simulink model "power_V2G_GA"  (R2015a)
settings: Solver=ode23tb  SolverMode=SingleTasking  StartTime=0.0  StopTime=24*60*60  RelTol=1e-4  AbsTol=1e-2
PreLoadFcn:
  | % Load Data and Parameters used by the model:
  | load power_V2G.mat
  | to=0.1;
undefined symbols (not defined in the file or in its folder): A, B, C, D1, Dd, Delta, Init, j, V2G
libraries: powerlib x54, simulink x19, simulink_extras x6, sps_avr x1, V2Glib x1, powerlib_meascontrol x1
(part 1 of 3)
Description:
  | Copyright 2008-2015 The MathWorks, Inc.
settings Model: SimulationMode=accelerator  CovSFcnEnable=off  ExtModeTrigDuration=100  Creator=MathWorks  LastModifiedBy=lenovo
settings SolverCC: MaxConsecutiveMinStep=1e6  ZeroCrossAlgorithm=Adaptive
settings OptimizationCC: BlockReduction=off  BooleanDataType=off
settings DebuggingCC: SaveWithParameterizedLinksMsg=none  UnderspecifiedInitializationDetection=Classic  MergeDetectMultiDrivingBlocksExec=none  SignalResolutionControl=TryResolveAllWithWarning
settings HardwareCC: TargetUnknown=on

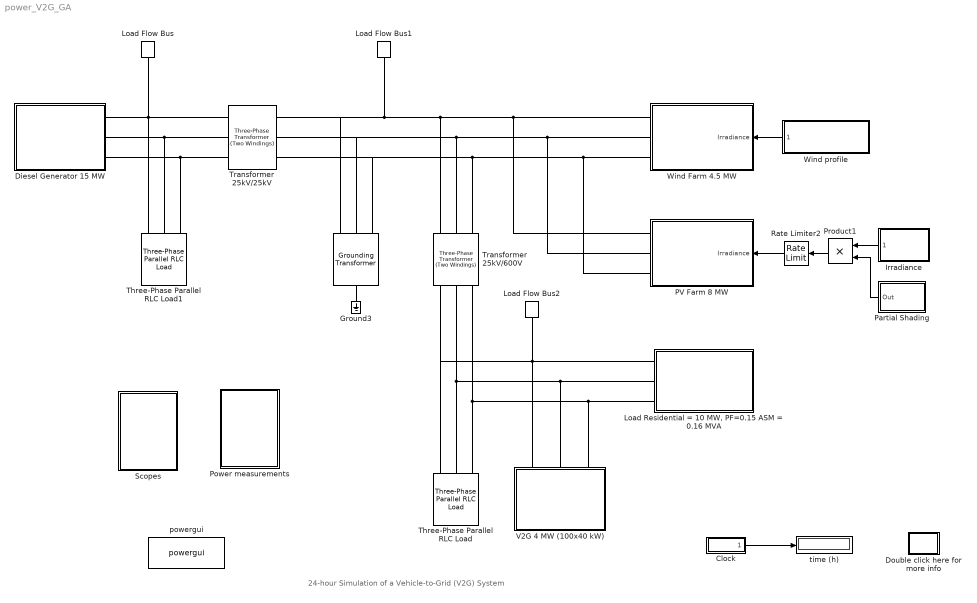
== system power_V2G_GA ==
  note: 24-hour Simulation of a Vehicle-to-Grid (V2G) System
  " " : powerlib/Elements/Grounding Transformer   UNITS=pu  NominalPower="[10e6   60]"  NominalVoltage=25e3  ZeroSequenceImpedance_pu=[0.00083333 9.4248]  MagnetizationBranch_pu=[5000 6283.2]  ZeroSequenceImpedance_SI=[0.25 7.5]  MagnetizationBranch_SI=[31250 31250]  Measurements=None
  Clock : Subsystem
  Diesel Generator 15 MW : Subsystem
      mask Display: image(imread('diesel.jpg'))
  Double click here for more info : Subsystem
      settings: OpenFcn=showdemo(bdroot(gcb))
      mask Display: disp('?')
  Ground3 : powerlib/Elements/Ground  LConnTagsString=a
  Irradiance : Subsystem
      mask init:
      | load power_V2G
      mask Display: plot(V2G.IRRADIANCE.time,V2G.IRRADIANCE.SUN)
  "Load Residential = 10 MW, PF=0.15 ASM = 0.16 MVA " : Subsystem
      mask Display: image(imread('load.jpg'))
  Load Flow Bus : powerlib/Measurements/Load Flow Bus  LConnTagsString=a  ID=BUS_1  Vbase=25e3  Vref=1  Vangle=0  VLF=1  angleLF=0
      settings: AttributesFormatString=%<ID>\n%<Vbase>V\n%<VLF>pu\n%<angleLF>deg.
  Load Flow Bus1 : powerlib/Measurements/Load Flow Bus  LConnTagsString=a  ID=BUS_2  Vbase=25e3  Vref=1  Vangle=0  VLF=0.9783  angleLF=-0.1322
      settings: AttributesFormatString=%<ID>\n%<Vbase>V\n%<VLF>pu\n%<angleLF>deg.
  Load Flow Bus2 : powerlib/Measurements/Load Flow Bus  LConnTagsString=a  ID=BUS_3  Vbase=1e3  Vref=1  Vangle=0  VLF=0.9583  angleLF=-3.174
      settings: AttributesFormatString=%<ID>\n%<Vbase>V\n%<VLF>pu\n%<angleLF>deg.
  PV Farm 8 MW : Subsystem  mask{eff=10, area=8e4}
      mask prompts: eff "Efficiency (%)"; area "Area (m^2)"
      mask help: The product of the effeciency, the area covered by the Pv farm and the irradiance in w/m2 will give you the power generate by the PV farm
      mask DialogControl DescGroupVar Prompt: PV farm
      mask DialogControl DescTextVar Prompt: The product of the efficiency, the area covered by the PV farm and the irradiance in W/m2 will give you the power generated by the PV farm.
      mask Display: image(imread('panel.jpg'))
  Partial Shading : Subsystem  mask(Signal Disturbance){Hour=12, Minute=0, Second=0, Duration=5*60, Factor=0.7}
      mask prompts: Duration "Duration (s):"
      mask help: Within the specified time range defined by Start and Duration parameters, output is set to 'Factor'. Outside the specified time range output is kept at 1.0.
      mask init:
      | T2=(Hour-1)*60*60;    % Hour in seconds
      | T3=(Minute-1)*60;  % Minute in seconds
      | Ton=T2+T3+(Second-1);    % Beginning of fault (s)
      | Toff=Ton+Duration; % End of fault (s)
      mask TypeOptions Hour: 0 |      1 |      2 |      3 |      4 |      5 |      6 |      7 |      8 |      9 |     10 |     11 |     12 |     13 |     14 |     15 |     16 |     17 |     18 |     19 |     20 |     21 |     22 |     23
      mask TypeOptions Minute: 0 |      1 |      2 |      3 |      4 |      5 |      6 |      7 |      8 |      9 |     10 |     11 |     12 |     13 |     14 |     15 |     16 |     17 |     18 |     19 |     20 |     21 |     22 |     23 |     24 |     25 |     26 |     27 |     28 |     29 |     30 |     31 |     32 |     33 |     34 |     35 |     36 |     37 |     38 |     39 |     40 |     41 |     42 |     43 |     44 |     45 |     46 |     47 |     48 |     49 |     50 |     51 |     52 |     53 |     54 |     55 |     56 |     57 |     58 |     59
      mask TypeOptions Second: 0 |      1 |      2 |      3 |      4 |      5 |      6 |      7 |      8 |      9 |     10 |     11 |     12 |     13 |     14 |     15 |     16 |     17 |     18 |     19 |     20 |     21 |     22 |     23 |     24 |     25 |     26 |     27 |     28 |     29 |     30 |     31 |     32 |     33 |     34 |     35 |     36 |     37 |     38 |     39 |     40 |     41 |     42 |     43 |     44 |     45 |     46 |     47 |     48 |     49 |     50 |     51 |     52 |     53 |     54 |     55 |     56 |     57 |     58 |     59
      mask DialogControl Control2 Prompt: Start:
  Power measurements : Subsystem
  Product1 : Product
  Rate Limiter2 : RateLimiter  RisingSlewLimit=1e4  FallingSlewLimit=-1e4  SampleTimeMode=inherited
  "Scopes " : Subsystem
  Three-Phase Parallel RLC Load : powerlib/Elements/Three-Phase Parallel RLC Load  LConnTagsString=A|B|C  Configuration=Y (grounded)  NominalVoltage=(1000)*0.958281  NominalFrequency=60  ActivePower=1e3  InductivePower=0  CapacitivePower=0  Measurements=None  LoadType=constant PQ
  Three-Phase Parallel RLC Load1 : powerlib/Elements/Three-Phase Parallel RLC Load  LConnTagsString=A|B|C  Configuration=Y (grounded)  NominalVoltage=(25000)*1  NominalFrequency=60  ActivePower=1e3  InductivePower=0  CapacitivePower=0  Measurements=None  LoadType=constant PQ
  Transformer 25kV/25kV : powerlib/Elements/Three-Phase Transformer (Two Windings)  Winding1Connection=Yg  Winding2Connection=Yg  CoreType=Three single-phase transformers  SetSaturation=off  Hysteresis=off  DataFile='hysteresis'  SetInitialFlux=off  Measurements=None  UNITS=pu  NominalPower=[ 20e6 , 60 ]  Winding1=[25e3 , 0.002 , 0.08 ]  Winding2=[ 25e3 , 0.002 , 0.08 ]  Rm=500  Lm=500  L0=0.5  Saturation=[ 0,0 ; 0.0024,1.2 ; 1.0,1.52 ]  InitialFluxes=[ 0.8 , -0.8 , 0.7 ]  MoreParameters=off  BreakLoop=off  DataType=off  TransfoNumber=1
  Transformer 25kV/600V : powerlib/Elements/Three-Phase Transformer (Two Windings)  Winding1Connection=Yg  Winding2Connection=Yg  CoreType=Three single-phase transformers  SetSaturation=off  Hysteresis=off  DataFile='hysteresis'  SetInitialFlux=off  Measurements=None  UNITS=pu  NominalPower=[ 20e6 , 60 ]  Winding1=[25e3 , 0.002 , 0.08 ]  Winding2=[ 600 , 0.002 , 0.08 ]  Rm=500  Lm=500  L0=0.5  Saturation=[ 0,0 ; 0.0024,1.2 ; 1.0,1.52 ]  InitialFluxes=[ 0.8 , -0.8 , 0.7 ]  MoreParameters=off  BreakLoop=off  DataType=off  TransfoNumber=1
  V2G 4 MW (100x40 kW) : Subsystem  mask{nomPower=20*2, capacity=85, eff=90, enable=on, regGain=[2 4e3], cars1=35, cars2=25, cars3=10, cars4=20, cars5=10}
      mask prompts: nomPower "Rated power (kW)"; capacity "Rated capacity (kWh)"; eff "System efficiency (%)"; enable "V2G on"; regGain "Regulator gain [Kp Ki]"; cars1 "Number of cars  (profile 1)"; cars2 "Number of cars  (profile 2)"; cars3 "Number of cars  (profile 3)"; cars4 "Number of cars  (profile 4)"; cars5 "Number of cars  (profile 5)"
      mask DialogControl DescGroupVar Prompt: V2G
      mask DialogControl DescTextVar Prompt: Models a generic aggregation of electric vehicles. The model has 5 different profiles that can be modified under the mask by changing the plug and the state of charge lookup tables of each profile. The user can set the number of vehicles following each type of profile. The rated capacity, the rated power and the efficiency of the power converter can also be decided by the user. See the example documentation for information about various user profiles.
      mask Display: image(imread('EV.jpg'))
  Wind Farm 4.5 MW : Subsystem  mask{nomPower=4.5, nomwind=13.5, maxwind=15}
      mask prompts: nomPower "Nominal power (MW)"; nomwind "Nominal wind speed (m/s)"; maxwind "Maximal wind speed (m/s)"
      mask DialogControl DescGroupVar Prompt: Wind farm
      mask DialogControl DescTextVar Prompt: The simplified wind farm model presented here generates power using a linear relationship between the nominal wind speed and nominal power. When the wind speed reaches the maximal value, the wind farm trips from the grid. When the wind speed is between the nominal speed and the maximal value, the power is fixed to 1 p.u.
      mask Display: image(imread('windfarm.jpg'))
  Wind profile : Subsystem
      mask init:
      | load power_V2G
      mask Display: plot(V2G.WINDTURBINE.time,V2G.WINDTURBINE.wind)
  powergui : powerlib/powergui  Priority=1  SimulationMode=Phasor  SolverType=Tustin  SampleTime=50e-6  frequency=60  SPID=off  DisableSnubberDevices=off  DisableRonSwitches=off  DisableVfSwitches=off  SwTol=0  DisplayEquations=off  Interpol=off  methode=off  Ts=100  FunctionMessages=off  echomessages=off  HookPort=off  EnableUseOfTLC=off  x0status=blocks  frequencyindice=60  Pbase=10e6  ErrMax=0.0001  Iterations=50  UnitsV=kV  UnitsW=MW  buscounter=0  RestoreLinks=warning  ResistiveCurrentMeasurement=off  Frange=[0:2:500]  Ylog=off  Xlog=on  ShowGrid=off  save=off  variable=ZData  structure=0  ZoomFFT=off  StartTime=0.0  cycles=1  DisplayStyle=1  fundamental=60  FreqAxis=off  MaxFrequency=1000  frequencyindicesteady=1  RmsSteady=1  display=off
  time (h) : Display
      settings: Format=bank
  wires:
  Irradiance/1(" ") -> Product1/1
  Product1/1 -> Rate Limiter2/1
  Wind profile/1(" ") -> Wind Farm 4.5 MW/1(Irradiance)
  Partial Shading/1(Out) -> Product1/2
  Rate Limiter2/1 -> PV Farm 8 MW/1(Irradiance)
  Clock/1(" ") -> time (h)/1
  connections:
  "Load Residential = 10 MW, PF=0.15 ASM = 0.16 MVA "/LConn3 -- V2G 4 MW (100x40 kW)/LConn3 -- Three-Phase Parallel RLC Load/LConn3 -- Transformer 25kV/600V/RConn3
  Transformer 25kV/600V/LConn3 -- " "/LConn3 -- Transformer 25kV/25kV/RConn3 -- PV Farm 8 MW/RConn3 -- Wind Farm 4.5 MW/RConn3
  " "/RConn1 -- Ground3/LConn1
  Load Flow Bus/LConn1 -- Transformer 25kV/25kV/LConn1 -- Diesel Generator 15 MW/RConn1 -- Three-Phase Parallel RLC Load1/LConn1
  "Load Residential = 10 MW, PF=0.15 ASM = 0.16 MVA "/LConn1 -- Load Flow Bus2/LConn1 -- V2G 4 MW (100x40 kW)/LConn1 -- Three-Phase Parallel RLC Load/LConn1 -- Transformer 25kV/600V/RConn1
  "Load Residential = 10 MW, PF=0.15 ASM = 0.16 MVA "/LConn2 -- V2G 4 MW (100x40 kW)/LConn2 -- Three-Phase Parallel RLC Load/LConn2 -- Transformer 25kV/600V/RConn2
  Transformer 25kV/600V/LConn1 -- Transformer 25kV/25kV/RConn1 -- " "/LConn1 -- Load Flow Bus1/LConn1 -- Wind Farm 4.5 MW/RConn1 -- PV Farm 8 MW/RConn1
  Transformer 25kV/600V/LConn2 -- " "/LConn2 -- Transformer 25kV/25kV/RConn2 -- PV Farm 8 MW/RConn2 -- Wind Farm 4.5 MW/RConn2
  Transformer 25kV/25kV/LConn3 -- Diesel Generator 15 MW/RConn3 -- Three-Phase Parallel RLC Load1/LConn3
  Transformer 25kV/25kV/LConn2 -- Diesel Generator 15 MW/RConn2 -- Three-Phase Parallel RLC Load1/LConn2

== system power_V2G_GA/Clock ==
  Clock : Clock
  Gain : Gain  Gain=1/(60*60)
  " " : Outport
  wires:
  Gain/1 -> " "/1
  Clock/1 -> Gain/1

== system power_V2G_GA/Diesel Generator 15 MW ==
  " Load Measurements" : powerlib/Measurements/Three-Phase V-I Measurement  VoltageMeasurement=phase-to-ground  SetLabelV=on  LabelV=Vabc1  Vpu=off  VpuLL=off  CurrentMeasurement=yes  SetLabelI=on  LabelI=Iabc1  Ipu=off  Pbase=2*1.5e6/0.9  Vbase=25e3  OutputType=Complex  PhasorSimulation=on  PSBequivalent=0
  Bus Selector : BusSelector  OutputSignals="dq0 components.Stator voltage  vq (pu),dq0 components.Stator voltage  vd (pu),Mechanical.Rotor speed  wm  (pu)"
  Constant1 : Constant
  Constant2 : Constant
  Diesel Engine Governor : Subsystem  mask(Diesel Engine & Governor){K=29, Tr=[0.01 0.02 0.2], Ta=[0.25 0.009 0.0384], Tlim=[0 1.1], Td=0.024, Pm0=0.1361}
      mask prompts: K "Regulator gain K:"; Tr "Regulator time constants [T1 T2 T3 ] (s) :"; Ta "Actuator time constants [T4 T5 T6] (s) :"; Tlim "Torque limits [Tmin Tmax] (pu) :"; Td "Engine time delay Td (s) :"; Pm0 "Initial value of mechanical power  Pm0 (pu) :"
      mask help:
      | This block implements a diesel engine and governor system:
      | 1st and 2nd inputs: Desired and actual speed (pu)
      | Output: Diesel engine mechanical power.Motor inertia should be combined with generator.
      | Controller transfer function:
      |      Hc=K.(1+T3.s)/(1+T1.s+T1.T2.s^2)
      | Actuator transfer function :
      |      Ha= (1+T4.s) / [ (s (1+T5.s)(1+T6.s) ]
      | Motor :
      |      Time delay Td
      |
      | (See reference in Tutorial Session 5)
  Excitation System : sps_avr/Excitation System  tr=20e-3  reg=[ 300, 0.001 ]  exc=[ 1, 0 ]  tgr=[ 0, 0 ]  damp=[ 0.001, 0.1 ]  sat=[ 0, 0 ]  lim=[ -11.5, 11.5, 0 ]  v0=[1 1.2473]
  Ground : Ground
  Rotor speed (p.u.) : Scope
      settings: TimeRange=86400  YMin=0.9955  YMax=1.005  SaveName=wm1
  Synchronous Machine pu Standard : powerlib/Machines/Synchronous Machine pu Standard  PresetModel=No  MechanicalLoad=Mechanical power Pm  ShowDetailedParameters=on  RotorType=Salient-pole  Units=per unit standard parameters  MeasurementBus=off  NominalParameters="[ 15E6  25e3   60]"  Reactances1=[ 1.81, 0.3, 0.23, 1.76, 0.65, 0.25, 0.15 ]  Reactances2="[ 1.305, 0.296, 0.252, 0.474,  0.243,  0.18 ]"  dAxisTimeConstants=Open-circuit  qAxisTimeConstants=Short-circuit  TimeConstants1="[ 4.4849  0.0681  0.1  ]"  TimeConstants2=[ 8.0, 0.03, 1.0, 0.07 ]  TimeConstants3="[  4.49  0.0681  0.0513  ]"  TimeConstants4=[ 8.0, 0.03, 0.3371, 0.0295 ]  TimeConstants5=[ 1.01, 0.053, 0.1 ]  TimeConstants6=[ 1.3201, 0.023, 1.0, 0.07 ]  TimeConstants7=[0.012 0.003 0.003]  TimeConstants8=[ 1.3201, 0.0231, 0.3371, 0.0295 ]  StatorResistance=0.003  Mechanical=[3.7 0 1 ]  PolePairs=20  InitialConditions=[0 -86.6365 0.2279 0.2279 0.2279 -53.3785 -173.379 66.6215 1.24735]  SetSaturation=off  Saturation=[0.6404,0.7127,0.8441,0.9214,0.9956,1.082,1.19,1.316,1.457;0.7,0.7698,0.8872,0.9466,0.9969,1.046,1.1,1.151,1.201]  LoadFlowParameters=[1,0,0,0,0]  TsPowergui=0  TsBlock=-1  IterativeModel=Trapezoidal non iterative  BusType=swing  Pref=0  Qref=0  Qmin=-inf  Qmax=inf  PLF=0  QLF=0
  A : PMIOPort  Port=1  Side=Right
  B : PMIOPort  Port=2  Side=Right
  C : PMIOPort  Port=3  Side=Right
  tag scope: wm=global
  wires:
  Bus Selector/3 -> Diesel Engine Governor/2(w (pu)), Rotor speed (p.u.)/1, [wm]  "<Rotor speed  wm  (pu)>"
  Constant1/1 -> Diesel Engine Governor/1(wref (pu))
  Diesel Engine Governor/1(Pmec (pu)) -> Synchronous Machine pu Standard/1
  Excitation System/1 -> Synchronous Machine pu Standard/2
  Constant2/1 -> Excitation System/1
  Bus Selector/2 -> Excitation System/2  "<Stator voltage  vd (pu)>"
  Bus Selector/1 -> Excitation System/3  "<Stator voltage  vq (pu)>"
  Synchronous Machine pu Standard/1 -> Bus Selector/1
  Ground/1 -> Excitation System/4
  connections:
  " Load Measurements"/RConn1 -- A/RConn1
  C/RConn1 -- " Load Measurements"/RConn3
  B/RConn1 -- " Load Measurements"/RConn2
  Synchronous Machine pu Standard/RConn3 -- " Load Measurements"/LConn3
  Synchronous Machine pu Standard/RConn2 -- " Load Measurements"/LConn2
  Synchronous Machine pu Standard/RConn1 -- " Load Measurements"/LConn1

== system power_V2G_GA/Double click here for more info ==

== system power_V2G_GA/Irradiance ==
  1-D Lookup IRRADIANCE Table : Lookup_n-D  NumberOfTableDimensions=1  BreakpointsForDimension1=V2G.IRRADIANCE.time  BeginIndexSearchUsingPreviousIndexResult=on  Table=V2G.IRRADIANCE.SUN  InternalRulePriority=Speed  RndMeth=Simplest  InputSameDT=on
  Add : Sum
  Clock : Clock
  Constant1 : Constant
  Second-->Hour : Gain  Gain=1/(60*60)
  " " : Outport
  wires:
  Constant1/1 -> Add/2
  Add/1 -> 1-D Lookup IRRADIANCE Table/1  "Hour of the day"
  1-D Lookup IRRADIANCE Table/1 -> " "/1
  Clock/1 -> Second-->Hour/1
  Second-->Hour/1 -> Add/1

== system power_V2G_GA/Load Residential = 10 MW, PF=0.15 ASM = 0.16 MVA  ==
  " ASM Measurements" : powerlib/Measurements/Three-Phase V-I Measurement  VoltageMeasurement=phase-to-ground  SetLabelV=on  LabelV=Vasm  Vpu=off  VpuLL=off  CurrentMeasurement=yes  SetLabelI=on  LabelI=Iasm  Ipu=off  Pbase=2*1.5e6/0.9  Vbase=25e3  OutputType=Complex  PhasorSimulation=on  PSBequivalent=0
  " Load Measurements" : powerlib/Measurements/Three-Phase V-I Measurement  VoltageMeasurement=phase-to-ground  SetLabelV=on  LabelV=Vload  Vpu=off  VpuLL=off  CurrentMeasurement=yes  SetLabelI=on  LabelI=Iload  Ipu=off  Pbase=2*1.5e6/0.9  Vbase=25e3  OutputType=Complex  PhasorSimulation=on  PSBequivalent=0
  Asynchronous Machine (customized) : V2Glib/Asynchronous Machine (custom)  RotorType=Squirrel-cage  PresetModel=No  MechanicalLoad=Torque Tm  ShowDetailedParameters=on  ReferenceFrame=Rotor  Units=pu  MeasurementBus=on  NominalParameters=[1.5e+05 600 60]  Stator=[0.01117 0.04832]  Rotor=[0.006 0.04832]  Cage1=[0.01909 0.0397]  Cage2=[0.01909 0.0397]  Lm=2.424  Mechanical=[0.3096 0.01511 2]  PolePairs=2  InitialConditions=[1 0 0 0 0 0 0 0]  SimulateSaturation=off  Saturation="[0.212,0.4201,0.8125,1.0979,1.4799,2.2457,3.2586,4.5763,6.4763 ;   0.5,0.7,0.9,1,1.1,1.2 ,1.3,1.4,1.5]"  LoadFlowParameters=0  TsPowergui=0  TsBlock=-1  IterativeModel=Trapezoidal non iterative  Pmec=2e6
  Gain : Gain  Gain=1.492e5
  Gain1 : Gain  Gain=1.018/(0.9825^2)
  Math Function : Math  Operator=square  SaturateOnIntegerOverflow=on
  P electric : Display
  Product : Product
  Rate Limiter2 : RateLimiter  RisingSlewLimit=1e4  FallingSlewLimit=-1e4  SampleTimeMode=inherited
  Residential Load : Subsystem  mask{nomPower=10, PF=0.95, timestep=60, datas=V2G.CONSUMPTION}
      mask prompts: nomPower "Nominal Power (MW)"; PF "Power factor"; timestep "Timestep (minutes)"; datas "Consumption datas"
      mask DialogControl DescGroupVar Prompt: Load profile
      mask DialogControl DescTextVar Prompt: The load profile allows you to fix a nominal power and and a power factor. It is also needed to specify the timestep used for the consumption datas. Finally, a vector expresses the consumption profile. It has to be expressed in per unit. It is imperative that the length of the vector fits with the timestep used.
      mask Display: image(imread('Residential.jpg'))
  Rotor speed (p.u.) : Display
  Te(p.u.) : Display
  Three-Phase Breaker2 : powerlib/Elements/Three-Phase Breaker  InitialState=open  SwitchA=on  SwitchB=on  SwitchC=on  SwitchTimes=[ 3*3600]  External=off  BreakerResistance=0.001  SnubberResistance=1e6  SnubberCapacitance=inf  Measurements=None
  Three-Phase Fault : powerlib/Elements/Three-Phase Fault  InitialStates=0  FaultA=off  FaultB=off  FaultC=off  GroundFault=on  SwitchTimes=[4*3600 4*3600+100]  External=off  SwitchStatus=NaN  FaultResistance=0.001  GroundResistance=0.01  SnubberResistance=1e6  SnubberCapacitance=inf  Measurements=None
  A : PMIOPort  Port=1  Side=Left
  B : PMIOPort  Port=2  Side=Left
  C : PMIOPort  Port=3  Side=Left
  wires:
  Gain1/1 -> Rate Limiter2/1
  Asynchronous Machine (customized)/1 -> Rotor speed (p.u.)/1, Product/1, Math Function/1
  Asynchronous Machine (customized)/2 -> Product/2, Te(p.u.)/1
  Product/1 -> Gain/1
  Gain/1 -> P electric/1
  Rate Limiter2/1 -> Asynchronous Machine (customized)/1
  Math Function/1 -> Gain1/1
  connections:
  " Load Measurements"/LConn3 -- Residential Load/LConn3
  " Load Measurements"/LConn2 -- Residential Load/LConn2
  " Load Measurements"/LConn1 -- Residential Load/LConn1
  " ASM Measurements"/RConn2 -- " Load Measurements"/RConn2 -- B/RConn1
  " ASM Measurements"/RConn3 -- " Load Measurements"/RConn3 -- C/RConn1
  " Load Measurements"/RConn1 -- A/RConn1 -- " ASM Measurements"/RConn1
  Asynchronous Machine (customized)/LConn2 -- Three-Phase Fault/LConn2 -- Three-Phase Breaker2/LConn2
  Asynchronous Machine (customized)/LConn3 -- Three-Phase Breaker2/LConn3 -- Three-Phase Fault/LConn3
  Three-Phase Breaker2/RConn1 -- " ASM Measurements"/LConn1
  Three-Phase Breaker2/RConn2 -- " ASM Measurements"/LConn2
  Three-Phase Breaker2/RConn3 -- " ASM Measurements"/LConn3
  Three-Phase Breaker2/LConn1 -- Three-Phase Fault/LConn1 -- Asynchronous Machine (customized)/LConn1

== system power_V2G_GA/PV Farm 8 MW ==
  Irradiance : Inport
  Irradiance data : Subsystem
  PV Farm : Subsystem
  VabcPV : powerlib/Measurements/Three-Phase V-I Measurement  VoltageMeasurement=phase-to-ground  SetLabelV=on  LabelV=VabcPV  Vpu=off  VpuLL=off  CurrentMeasurement=yes  SetLabelI=on  LabelI=IabcPV  Ipu=off  Pbase=2*1.5e6/0.9  Vbase=25e3  OutputType=Complex  PhasorSimulation=on  PSBequivalent=0
  A : PMIOPort  Port=1  Side=Right
  B : PMIOPort  Port=2  Side=Right
  C : PMIOPort  Port=3  Side=Right
  wires:
  Irradiance data/1(Out1) -> PV Farm/1(P)
  Irradiance/1 -> Irradiance data/1("Data ")
  connections:
  B/RConn1 -- VabcPV/RConn2
  VabcPV/LConn2 -- PV Farm/RConn2
  A/RConn1 -- VabcPV/RConn1
  VabcPV/RConn3 -- C/RConn1
  PV Farm/RConn1 -- VabcPV/LConn1
  VabcPV/LConn3 -- PV Farm/RConn3

== system power_V2G_GA/Partial Shading ==
  Add : Sum
  Clock : Clock
  Compare To Constant : simulink/Logic and Bit Operations/Compare To Constant  relop=>=  const=Ton  OutDataTypeStr=boolean
  Compare To Constant1 : simulink/Logic and Bit Operations/Compare To Constant  relop=<  const=Toff  OutDataTypeStr=boolean
  Constant : Constant  Value=Factor
  Logical Operator : Logic  AllPortsSameDT=off  OutDataTypeStr=float('double')
  Logical Operator1 : Logic  Operator=NOT  AllPortsSameDT=off  OutDataTypeStr=float('double')
  Product : Product
  Out : Outport
  wires:
  Add/1 -> Out/1
  Product/1 -> Add/2
  Constant/1 -> Product/2
  Compare To Constant/1 -> Logical Operator/1
  Clock/1 -> Compare To Constant1/1, Compare To Constant/1
  Compare To Constant1/1 -> Logical Operator/2
  Logical Operator/1 -> Logical Operator1/1, Product/1
  Logical Operator1/1 -> Add/1

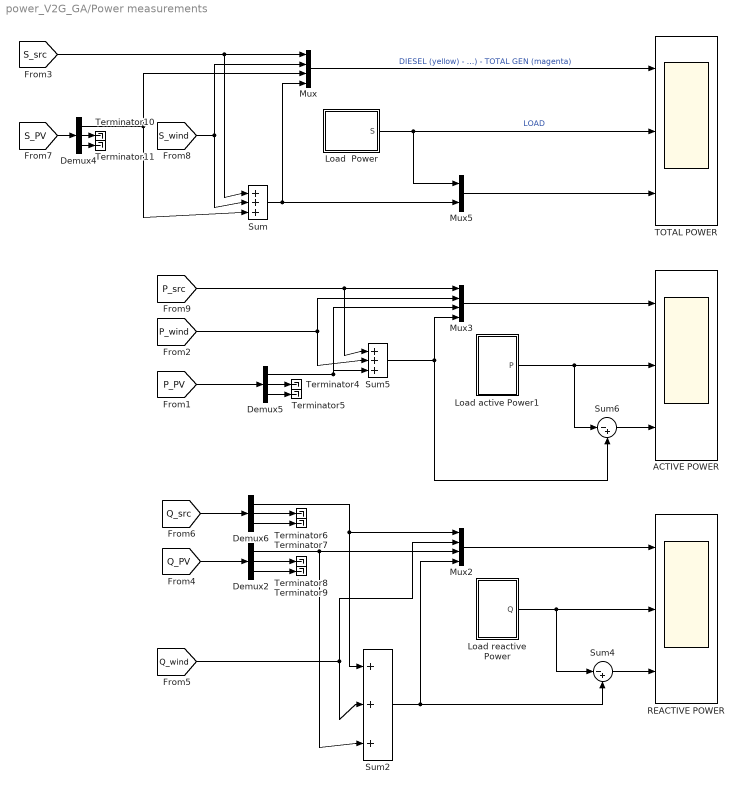
== system power_V2G_GA/Power measurements ==
  ACTIVE POWER : Scope  NumInputPorts=3
      settings: TimeRange=86394.68034477012  YMin=-1127645.502645526~0~0  YMax=14321145.12471653~14000000~194678.5071649832  SaveName=ScopeData9  Decimation=20
  Demux{2,4..6} (4 alike) : Demux  Outputs=3
  Load  Power : Subsystem
  Load active Power1 : Subsystem
  Load reactive Power : Subsystem
  Mux : Mux
  Mux2 : Mux
  Mux3 : Mux
  Mux5 : Mux  Inputs=2
  REACTIVE POWER : Scope  NumInputPorts=3
      settings: TimeRange=86394.68034477012  YMin=-639880.9523809515~29417.73813057679~0  YMax=7141203.703703707~4200987.36115234~2993413.800705456  SaveName=ScopeData7  Decimation=20
  Sum : Sum  Inputs=|+++
  Sum2 : Sum  Inputs=|+++
  Sum4 : Sum  Inputs=|-+
  Sum5 : Sum  Inputs=|+++
  Sum6 : Sum  Inputs=|-+
  TOTAL POWER : Scope  NumInputPorts=3
      settings: TimeRange=86395.43113750442  YMin=0~0~123381.0870346278  YMax=16020911.12187349~14000000~16409684.57560659  SaveName=ScopeData5  Decimation=20
  Terminator{4..11} (8 alike) : Terminator
  wires:
  [Q_src] -> Demux6/1
  [S_src] -> Sum/1, Mux/1
  [S_wind] -> Mux/2, Sum/2
  Sum/1 -> Mux/4, Mux5/2
  Demux6/1 -> Sum2/1, Mux2/1
  [Q_wind] -> Mux2/2, Sum2/2
  Sum2/1 -> Sum4/2, Mux2/4
  Mux/1 -> TOTAL POWER/1  "DIESEL (yellow) - WIND (red) - PV FARM (green) - TOTAL GEN (magenta)"
  Mux2/1 -> REACTIVE POWER/1
  Sum4/1 -> REACTIVE POWER/3
  Mux5/1 -> TOTAL POWER/3
  Load  Power/1(S) -> TOTAL POWER/2, Mux5/1  "LOAD"
  [Q_PV] -> Demux2/1
  Demux2/1 -> Sum2/3, Mux2/3
  [S_PV] -> Demux4/1
  Demux4/2 -> Terminator10/1
  Demux4/3 -> Terminator11/1
  Demux4/1 -> Mux/3, Sum/3
  Load reactive Power/1("Q ") -> Sum4/1, REACTIVE POWER/2
  [P_wind] -> Sum5/2, Mux3/2
  [P_src] -> Sum5/1, Mux3/1
  Sum5/1 -> Sum6/2, Mux3/4
  Mux3/1 -> ACTIVE POWER/1
  Load active Power1/1(P) -> Sum6/1, ACTIVE POWER/2
  Sum6/1 -> ACTIVE POWER/3
  [P_PV] -> Demux5/1
  Demux5/1 -> Sum5/3, Mux3/3
  Demux5/2 -> Terminator4/1
  Demux5/3 -> Terminator5/1
  Demux6/2 -> Terminator6/1
  Demux6/3 -> Terminator7/1
  Demux2/2 -> Terminator8/1
  Demux2/3 -> Terminator9/1

== system power_V2G_GA/Scopes  ==
  note: Scopes related to production
  note: Scopes related to the consumption
  note: Scopes related to the V2G system
  ASM : Scope  NumInputPorts=5
      settings: TimeRange=86394.68034477012  YMin=383.346641994195~0~0~-279310.3448275863~-231272.2948870416  YMax=518.2077387266461~464.9227110582633~270214.030915576~0~92152.19976218522  SaveName=ScopeData10  Decimation=20
  ASMdata : Subsystem
  Charge : Scope  NumInputPorts=5
      settings: YMin=449.78~0.00075~0.5~-0.95~-0.3  YMax=449.87~0.00135~0.95~-0.45~0.3  SaveName=ScopeData17  Decimation=20
  Charge data : Subsystem
  Load : Scope  NumInputPorts=5
      settings: TimeRange=86394.68034477012  YMin=395.7726844069046~6091.95402298851~4224137.931034483~-11810344.8275862~-4000000  YMax=499.0979539956536~18045.97701149426~12500000~-3706896.551724136~-655172.4137931094  Decimation=20
  "Load data " : Subsystem
  PV Farm : Scope  NumInputPorts=5
      settings: TimeRange=86394.68034477012  YMin=18282.00607471011~0~0~-124521.0727969295~-229885.0574712642  YMax=20769.83390958213~150~4430232.558139537~4752609.327520147~172413.7931034481  SaveName=ScopeData14  Decimation=20
  "PV farm data " : Subsystem
  Regulation : Scope  NumInputPorts=5
      settings: TimeRange=86394.68034477012  YMin=421.4094484724554~0~0~-5000000~-139204.545454545  YMax=494.7795494032165~6000~4000000~5000000~184659.0909090918  SaveName=ScopeData15  Decimation=20
  Regulation data : Subsystem
  Sequence Analyzer (Phasor) : powerlib_meascontrol/Measurements/Sequence Analyzer (Phasor)  seq=Positive Negative Zero
  Sequences : Scope  NumInputPorts=2
      settings: TimeRange=86394.68034477012  YMin=0~-200  YMax=3500~200  SaveName=ScopeData6  Decimation=20
  Source : Scope  NumInputPorts=5
      settings: TimeRange=86394.68034477012  YMin=19667.0693040594~0~0~0~0  YMax=20918.20386543416~400~14997637.78661004~12955761.02158985~8413549.565165743  SaveName=ScopeData2  Decimation=20
  Source data : Subsystem
  State of charge : Scope  NumInputPorts=5
      settings: TimeRange=86394.68034477012  YMin=-50~-50~-50~89.99500000000001~-100  YMax=100~100~100~90.00500000000001~100  SaveName=ScopeData16  Decimation=20
  Wind Farm : Scope  NumInputPorts=6
      settings: TimeRange=86394.68034477012  YMin=432.0011600969374~0~0~-746268.6567164138~-1305413.232345677~0  YMax=474.3252378462745~8134.328358208958~6532635.330808647~5000000~833147.6943640569~20  SaveName=ScopeData8  Decimation=20
  Wind farm data : Subsystem
  wires:
  Source data/5(Q src) -> Source/5  "Q_src"
  Source data/4(P src) -> Source/4  "P_src"
  Source data/3(S src) -> Source/3  "S_src"
  Source data/2(I src) -> Source/2  "I_src"
  Source data/1(V src) -> Source/1  "V_src"
  "Load data "/5(Q load) -> Load/5  "Q_load"
  "Load data "/1(V load) -> Load/1  "V_load"
  "Load data "/2(I load) -> Load/2  "I_load"
  "Load data "/3(S load) -> Load/3  "S_load"
  "Load data "/4(P load) -> Load/4  "P_load"
  Wind farm data/5(Q wind) -> Wind Farm/5  "Q_wind"
  Wind farm data/1(V wind) -> Wind Farm/1  "V_wind"
  Wind farm data/2(I wind) -> Wind Farm/2  "I_wind"
  Wind farm data/3(S wind) -> Wind Farm/3  "S_wind"
  Wind farm data/4(P wind) -> Wind Farm/4  "P_wind"
  Wind farm data/6(Wind) -> Wind Farm/6  "Wind"
  "PV farm data "/1(V PV) -> PV Farm/1  "V_PV"
  "PV farm data "/2(I PV) -> PV Farm/2  "I_PV"
  "PV farm data "/3(S PV) -> PV Farm/3  "S_PV"
  "PV farm data "/5(Q PV) -> PV Farm/5  "Q_PV"
  "PV farm data "/4(P PV) -> PV Farm/4  "P_PV"
  Regulation data/1(V reg) -> Regulation/1
  Regulation data/2(I reg) -> Regulation/2
  Regulation data/3(S reg) -> Regulation/3
  Regulation data/5(Q reg) -> Regulation/5
  Regulation data/4(P reg) -> Regulation/4
  Charge data/1(V charg) -> Charge/1
  Charge data/2(I charg) -> Charge/2
  Charge data/3(S charg) -> Charge/3
  Charge data/5(Q charg) -> Charge/5
  Charge data/4(P charg) -> Charge/4
  [SOCcars2] -> State of charge/2
  [SOCcars3] -> State of charge/3
  [SOCcars4] -> State of charge/4
  [SOCcars5] -> State of charge/5
  [SOCcars1] -> State of charge/1
  ASMdata/5(Q asm) -> ASM/5  "Q_asm"
  ASMdata/1(V asm) -> ASM/1  "V_asm"
  ASMdata/2(I asm) -> ASM/2  "I_asm"
  ASMdata/3(S asm) -> ASM/3  "S_asm"
  ASMdata/4(P asm) -> ASM/4  "P_asm"
  Sequence Analyzer (Phasor)/1 -> Sequences/1
  Sequence Analyzer (Phasor)/2 -> Sequences/2
  [Iasm] -> Sequence Analyzer (Phasor)/1

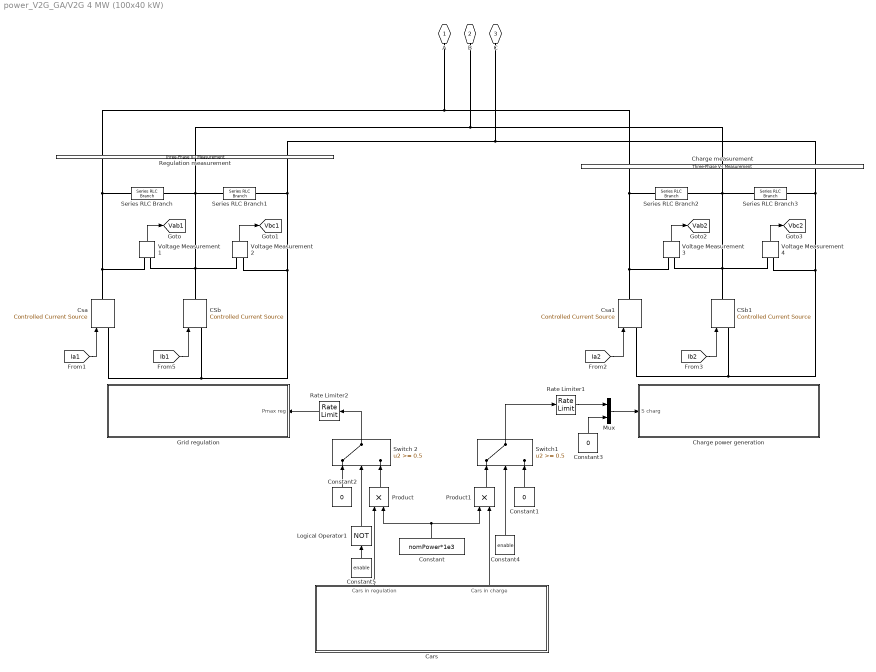
== system power_V2G_GA/V2G 4 MW (100x40 kW) ==
  " Charge measurement" : powerlib/Measurements/Three-Phase V-I Measurement  VoltageMeasurement=phase-to-ground  SetLabelV=on  LabelV=V_charg  Vpu=off  VpuLL=off  CurrentMeasurement=yes  SetLabelI=on  LabelI=I_charg  Ipu=off  Pbase=2*1.5e6/0.9  Vbase=25e3  OutputType=Complex  PhasorSimulation=on  PSBequivalent=0
  " Regulation measurement" : powerlib/Measurements/Three-Phase V-I Measurement  VoltageMeasurement=phase-to-ground  SetLabelV=on  LabelV=V_EV  Vpu=off  VpuLL=off  CurrentMeasurement=yes  SetLabelI=on  LabelI=I_EV  Ipu=off  Pbase=2*1.5e6/0.9  Vbase=25e3  OutputType=Complex  PhasorSimulation=on  PSBequivalent=0
  CSb : powerlib/Electrical Sources/Controlled Current Source  Initialize=on  Source_Type=AC  Amplitude=5604.181  Phase=(2.761-2*pi/3)*180/pi  Frequency=60  Measurements=Current
  CSb1 : powerlib/Electrical Sources/Controlled Current Source  Initialize=on  Source_Type=AC  Amplitude=5604.181  Phase=(2.761-2*pi/3)*180/pi  Frequency=60  Measurements=Current
  Cars : Subsystem
  Charge power generation : Subsystem
  Constant : Constant  Value=nomPower*1e3
  Constant1 : Constant  Value=0
  Constant2 : Constant  Value=0
  Constant3 : Constant  Value=0
  Constant4 : Constant  Value=enable
  Constant5 : Constant  Value=enable
  Csa : powerlib/Electrical Sources/Controlled Current Source  Initialize=on  Source_Type=AC  Amplitude=5604.181  Phase=2.761*180/pi  Frequency=60  Measurements=Current
  Csa1 : powerlib/Electrical Sources/Controlled Current Source  Initialize=on  Source_Type=AC  Amplitude=5604.181  Phase=2.761*180/pi  Frequency=60  Measurements=Current
  Grid regulation : Subsystem
  Logical Operator1 : Logic  Operator=NOT  AllPortsSameDT=off  OutDataTypeStr=boolean
  Mux : Mux  Inputs=2
  Product : Product
  Product1 : Product
  Rate Limiter1 : RateLimiter  RisingSlewLimit=1e4  FallingSlewLimit=-1e4  SampleTimeMode=inherited
  Rate Limiter2 : RateLimiter  RisingSlewLimit=1e4  FallingSlewLimit=-1e4  SampleTimeMode=inherited
  Series RLC Branch{,1..3} (4 alike) : powerlib/Elements/Series RLC Branch  LConnTagsString=__new0  RConnTagsString=__new0  BranchType=R  Resistance=1e6  Inductance=1e-3  SetiL0=off  InitialCurrent=0  Capacitance=1e-6  Setx0=off  InitialVoltage=0  Measurements=None
  Switch 2 : Switch  Threshold=0.5  ZeroCross=off
  Switch1 : Switch  Threshold=0.5  ZeroCross=off
  Voltage Measurement{1..4} (4 alike) : powerlib/Measurements/Voltage Measurement  PhasorSimulation=on  OutputType=Complex  PSBequivalent=0
  "A " : PMIOPort  Tag=PMCPort  Port=1  Side=Left
  B : PMIOPort  Tag=PMCPort  Port=2  Side=Left
  "C " : PMIOPort  Tag=PMCPort  Port=3  Side=Left
  tag scope: Vab1=global, Vab2=global, Vbc1=global, Vbc2=global
  wires:
  Voltage Measurement1/1 -> [Vab1]
  Voltage Measurement2/1 -> [Vbc1]
  [Ia1] -> Csa/1
  [Ib1] -> CSb/1
  Voltage Measurement3/1 -> [Vab2]
  Voltage Measurement4/1 -> [Vbc2]
  [Ia2] -> Csa1/1
  [Ib2] -> CSb1/1
  Constant/1 -> Product/2, Product1/1
  Constant3/1 -> Mux/2
  Mux/1 -> Charge power generation/1(S charg)
  Cars/1(Cars in regulation) -> Product/1
  Cars/2(" Cars in charge") -> Product1/2
  Constant2/1 -> Switch 2/1
  Switch 2/1 -> Rate Limiter2/1
  Product1/1 -> Switch1/1
  Constant1/1 -> Switch1/3
  Switch1/1 -> Rate Limiter1/1
  Product/1 -> Switch 2/3
  Constant5/1 -> Logical Operator1/1
  Constant4/1 -> Switch1/2
  Logical Operator1/1 -> Switch 2/2
  Rate Limiter1/1 -> Mux/1
  Rate Limiter2/1 -> Grid regulation/1(Pmax reg)
  connections:
  Series RLC Branch/LConn1 -- " Regulation measurement"/LConn1 -- Csa/RConn1 -- Voltage Measurement1/LConn1
  Voltage Measurement2/LConn2 -- Series RLC Branch1/RConn1 -- " Regulation measurement"/LConn3 -- Csa/LConn1 -- CSb/LConn1
  CSb/RConn1 -- Voltage Measurement1/LConn2 -- Voltage Measurement2/LConn1 -- Series RLC Branch/RConn1 -- " Regulation measurement"/LConn2 -- Series RLC Branch1/LConn1
  Voltage Measurement3/LConn1 -- Csa1/RConn1 -- Series RLC Branch2/LConn1 -- " Charge measurement"/LConn1
  Series RLC Branch3/RConn1 -- " Charge measurement"/LConn3 -- Voltage Measurement4/LConn2 -- Csa1/LConn1 -- CSb1/LConn1
  Series RLC Branch3/LConn1 -- Series RLC Branch2/RConn1 -- Voltage Measurement3/LConn2 -- CSb1/RConn1 -- Voltage Measurement4/LConn1 -- " Charge measurement"/LConn2
  " Regulation measurement"/RConn1 -- "A "/RConn1 -- " Charge measurement"/RConn1
  " Regulation measurement"/RConn2 -- " Charge measurement"/RConn2 -- B/RConn1
  " Charge measurement"/RConn3 -- " Regulation measurement"/RConn3 -- "C "/RConn1

== system power_V2G_GA/Wind Farm 4.5 MW ==
  Irradiance : Inport
  25 kV/ 575 V 6*2 MVA : powerlib/Elements/Three-Phase Transformer (Two Windings)  Winding1Connection=Yg  Winding2Connection=Delta (D1)  CoreType=Three single-phase transformers  SetSaturation=off  Hysteresis=off  DataFile='hysteresis'  SetInitialFlux=off  Measurements=None  UNITS=pu  NominalPower="[6*2e6  60]"  Winding1=[25e3 , 0.025/30 , 0.025]  Winding2=[ 575, 0.025/30 , 0.025]  Rm=500  Lm=inf  L0=0.5  Saturation=[ 0,0 ; 0.0024,1.2 ; 1.0,1.52 ]  InitialFluxes=[ 0.8 , -0.8 , 0.7 ]  MoreParameters=off  BreakLoop=off  DataType=off  TransfoNumber=0
  B575 (575 V) : powerlib/Measurements/Three-Phase V-I Measurement  VoltageMeasurement=phase-to-ground  SetLabelV=on  LabelV=Vabcwind  Vpu=off  VpuLL=off  CurrentMeasurement=yes  SetLabelI=on  LabelI=Iabcwind  Ipu=off  Pbase=6*1.5e6/0.9  Vbase=575  OutputType=Complex  PhasorSimulation=on  PSBequivalent=0
  Load 1kW : powerlib/Elements/Three-Phase Series RLC Load  LConnTagsString=A|B|C  Configuration=Y (grounded)  NominalVoltage=(575)*0.978785  NominalFrequency=60  ActivePower=1e3  InductivePower=0  CapacitivePower=0  Measurements=None  LoadType=constant PQ
  Load Flow Bus : powerlib/Measurements/Load Flow Bus  LConnTagsString=a  ID=BUS_575  Vbase=575  Vref=1  Vangle=0  VLF=0.9788  angleLF=-28.64
      settings: AttributesFormatString=%<ID>\n%<Vbase>V\n%<VLF>pu\n%<angleLF>deg.
  Three-Phase Source : powerlib/Electrical Sources/Three-Phase Source  Voltage=0  PhaseAngle=52.757  Frequency=60  InternalConnection=Yg  SpecifyImpedance=on  Resistance=0.8929  Inductance=16.58e-3  ShortCircuitLevel=100e6  BaseVoltage=25e3  XRratio=7  BusType=PV  Pref=6e6  Qref=0  Qmin=-inf  Qmax=inf
  Wind Farm : Subsystem
  Wind control : Subsystem
  A : PMIOPort  Port=1  Side=Right
  B : PMIOPort  Port=2  Side=Right
  C : PMIOPort  Port=3  Side=Right
  tag scope: wind=global
  wires:
  Wind control/1(Wind) -> Wind Farm/1("wind "), [wind]
  Irradiance/1 -> Wind control/1("wind ")
  connections:
  A/RConn1 -- 25 kV/ 575 V 6*2 MVA/LConn1
  B/RConn1 -- 25 kV/ 575 V 6*2 MVA/LConn2
  C/RConn1 -- 25 kV/ 575 V 6*2 MVA/LConn3
  B575 (575 V)/RConn1 -- Load 1kW/LConn1 -- 25 kV/ 575 V 6*2 MVA/RConn1
  B575 (575 V)/RConn2 -- Load 1kW/LConn2 -- 25 kV/ 575 V 6*2 MVA/RConn2
  B575 (575 V)/RConn3 -- Load 1kW/LConn3 -- 25 kV/ 575 V 6*2 MVA/RConn3
  Load Flow Bus/LConn1 -- Wind Farm/RConn3 -- Three-Phase Source/RConn3 -- B575 (575 V)/LConn3
  B575 (575 V)/LConn1 -- Wind Farm/RConn1 -- Three-Phase Source/RConn1
  B575 (575 V)/LConn2 -- Wind Farm/RConn2 -- Three-Phase Source/RConn2

== system power_V2G_GA/Wind profile ==
  1-D Lookup Table : Lookup_n-D  NumberOfTableDimensions=1  BreakpointsForDimension1=V2G.WINDTURBINE.time  BeginIndexSearchUsingPreviousIndexResult=on  Table=V2G.WINDTURBINE.wind  ExtrapMethod=Clip  UseLastTableValue=on  InternalRulePriority=Speed  RndMeth=Simplest  InputSameDT=on
  Add : Sum
  Clock : Clock
  Constant1 : Constant
  Second-->Hour : Gain  Gain=1/(60*60)
  " " : Outport
  wires:
  Second-->Hour/1 -> Add/1
  Add/1 -> 1-D Lookup Table/1
  Constant1/1 -> Add/2
  Clock/1 -> Second-->Hour/1
  1-D Lookup Table/1 -> " "/1

== system power_V2G_GA/Diesel Generator 15 MW/Diesel Engine Governor ==
  note: ACTUATOR
  wref (pu) : Inport
  w (pu) : Inport  Port=2
  CONTROL SYSTEM : TransferFcn  Numerator=([Tr(3) 1])  Denominator="([Tr(1)*Tr(2)  Tr(1) 1])"
  ENGINE Td : TransportDelay  DelayTime=Td  InitialOutput=Pm0
  Gain K : Gain  Gain=K  SaturateOnIntegerOverflow=on  OutDataTypeStr=Inherit: Same as input  ParamDataTypeStr=Inherit: Same as input
  Integrator : Integrator  InitialCondition=Pm0  LimitOutput=on  UpperSaturationLimit=Tlim(2)  LowerSaturationLimit=Tlim(1)
  Product : Product  SaturateOnIntegerOverflow=on  InputSameDT=on  OutDataTypeStr=Inherit: Same as first input
  Sum : Sum  Inputs=+-  SaturateOnIntegerOverflow=on  InputSameDT=on  OutDataTypeStr=Inherit: Same as first input
  TF1 : TransferFcn  Numerator=([Ta(1) 1])  Denominator=([Ta(2) 1])
  TF2 : TransferFcn  Numerator=1  Denominator=([Ta(3) 1])
  Pmec (pu) : Outport  InitialOutput=0
  wires:
  Gain K/1 -> TF1/1
  Sum/1 -> CONTROL SYSTEM/1
  CONTROL SYSTEM/1 -> Gain K/1
  TF1/1 -> TF2/1
  w (pu)/1 -> Product/2, Sum/2
  ENGINE Td/1 -> Product/1
  wref (pu)/1 -> Sum/1
  Product/1 -> Pmec (pu)/1
  TF2/1 -> Integrator/1
  Integrator/1 -> ENGINE Td/1  "Torque"

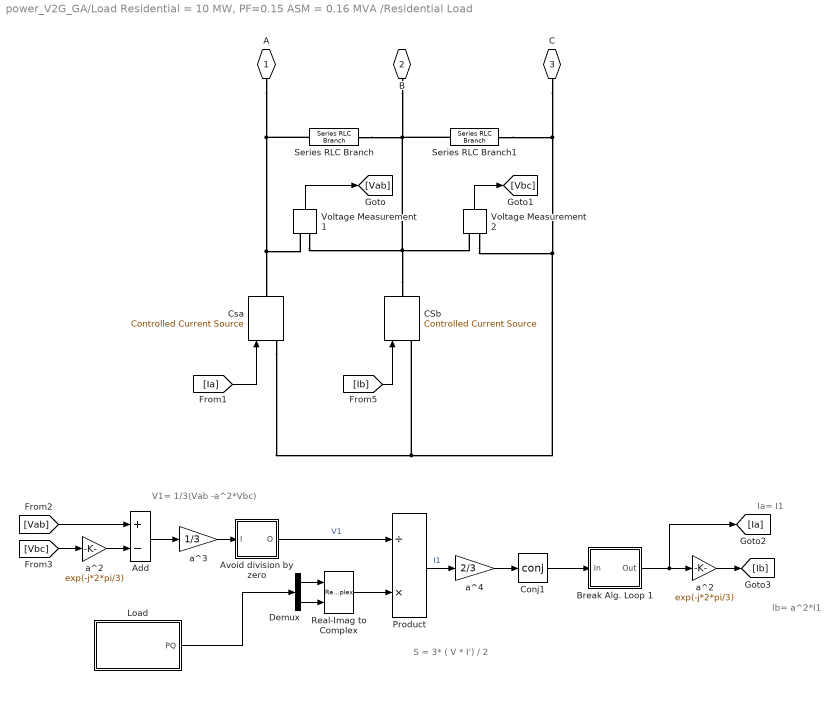
== system power_V2G_GA/Load Residential = 10 MW, PF=0.15 ASM = 0.16 MVA /Residential Load ==
  note: V1= 1/3(Vab -a^2*Vbc)
  note: S = 3* ( V * I') / 2
  note: Ia= I1
  note: Ib= a^2*I1
  Add : Sum  Inputs=+-
  Avoid division by zero : Subsystem
  Break Alg. Loop 1 : Subsystem
  CSb : powerlib/Electrical Sources/Controlled Current Source  Initialize=on  Source_Type=AC  Amplitude=9355.5  Phase=(2.751-2*pi/3)*180/pi  Frequency=60  Measurements=Current
  Conj1 : Math  Operator=conj  SaturateOnIntegerOverflow=on
  Csa : powerlib/Electrical Sources/Controlled Current Source  Initialize=on  Source_Type=AC  Amplitude=9355.5  Phase=2.751*180/pi  Frequency=60  Measurements=Current
  Demux : Demux  Outputs=2
  Load : Subsystem
  Product : Product  Inputs=/*  SaturateOnIntegerOverflow=on  InputSameDT=on  OutDataTypeStr=Inherit: Same as first input
  Real-Imag to Complex : RealImagToComplex
  Series RLC Branch : powerlib/Elements/Series RLC Branch  LConnTagsString=__new0  RConnTagsString=__new0  BranchType=R  Resistance=1e6  Inductance=1e-3  SetiL0=off  InitialCurrent=0  Capacitance=1e-6  Setx0=off  InitialVoltage=0  Measurements=None
  Series RLC Branch1 : powerlib/Elements/Series RLC Branch  LConnTagsString=__new0  RConnTagsString=__new0  BranchType=R  Resistance=1e6  Inductance=1e-3  SetiL0=off  InitialCurrent=0  Capacitance=1e-6  Setx0=off  InitialVoltage=0  Measurements=None
  Voltage Measurement1 : powerlib/Measurements/Voltage Measurement  PhasorSimulation=on  OutputType=Complex  PSBequivalent=0
  Voltage Measurement2 : powerlib/Measurements/Voltage Measurement  PhasorSimulation=on  OutputType=Complex  PSBequivalent=0
  a^2 : Gain  Gain=exp(-j*2*pi/3)  SaturateOnIntegerOverflow=on  OutDataTypeStr=Inherit: Same as input  ParamDataTypeStr=Inherit: Same as input
  "a^2 " : Gain  Gain=exp(-j*2*pi/3)  SaturateOnIntegerOverflow=on  OutDataTypeStr=Inherit: Same as input  ParamDataTypeStr=Inherit: Same as input
  a^3 : Gain  Gain=1/3  SaturateOnIntegerOverflow=on  OutDataTypeStr=Inherit: Same as input  ParamDataTypeStr=Inherit: Same as input
  a^4 : Gain  Gain=2/3  SaturateOnIntegerOverflow=on  OutDataTypeStr=Inherit: Same as input  ParamDataTypeStr=Inherit: Same as input
  A : PMIOPort  Tag=PMCPort  Port=1  Side=Left
  B : PMIOPort  Tag=PMCPort  Port=2  Side=Left
  C : PMIOPort  Tag=PMCPort  Port=3  Side=Left
  wires:
  Voltage Measurement1/1 -> [Vab]
  Voltage Measurement2/1 -> [Vbc]
  [Ia] -> Csa/1
  [Ib] -> CSb/1
  Real-Imag to Complex/1 -> Product/2
  Product/1 -> a^4/1  "I1"
  a^2/1 -> [Ib]
  a^3/1 -> Avoid division by zero/1(I)
  Add/1 -> a^3/1
  [Vab] -> Add/1
  [Vbc] -> "a^2 "/1
  "a^2 "/1 -> Add/2
  a^4/1 -> Conj1/1
  Demux/1 -> Real-Imag to Complex/1
  Demux/2 -> Real-Imag to Complex/2
  Load/1(PQ) -> Demux/1
  Avoid division by zero/1(O) -> Product/1  "V1"
  Conj1/1 -> Break Alg. Loop 1/1(In)
  Break Alg. Loop 1/1(Out) -> [Ia], a^2/1
  connections:
  Series RLC Branch/LConn1 -- A/RConn1 -- Csa/RConn1 -- Voltage Measurement1/LConn1
  Voltage Measurement2/LConn2 -- C/RConn1 -- Series RLC Branch1/RConn1 -- Csa/LConn1 -- CSb/LConn1
  CSb/RConn1 -- Voltage Measurement2/LConn1 -- Voltage Measurement1/LConn2 -- B/RConn1 -- Series RLC Branch1/LConn1 -- Series RLC Branch/RConn1

== system power_V2G_GA/PV Farm 8 MW/Irradiance data ==
  "Data " : Inport
  efficiency : Gain  Gain=eff/100
  m2 : Gain  Gain=area
  Out1 : Outport
  wires:
  m2/1 -> efficiency/1
  "Data "/1 -> m2/1
  efficiency/1 -> Out1/1

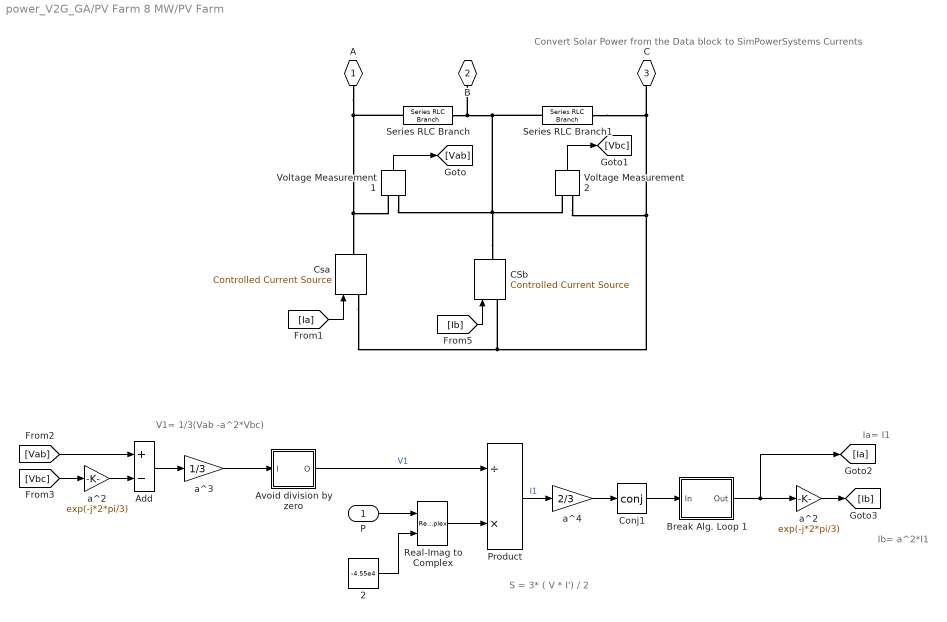
== system power_V2G_GA/PV Farm 8 MW/PV Farm ==
  note: Ib= a^2*I1
  note: Ia= I1
  note: S = 3* ( V * I') / 2
  note: V1= 1/3(Vab -a^2*Vbc)
  note: Convert Solar Power from the Data block to SimPowerSystems Currents
  P : Inport
  2 : Constant  Value=-4.55e4
  Add : Sum  Inputs=+-
  Avoid division by zero : Subsystem
  Break Alg. Loop 1 : Subsystem
  CSb : powerlib/Electrical Sources/Controlled Current Source  Initialize=on  Source_Type=AC  Amplitude=0  Phase=0  Frequency=60  Measurements=None
  Conj1 : Math  Operator=conj  SaturateOnIntegerOverflow=on
  Csa : powerlib/Electrical Sources/Controlled Current Source  Initialize=on  Source_Type=AC  Amplitude=0  Phase=0  Frequency=60  Measurements=None
  Product : Product  Inputs=/*  SaturateOnIntegerOverflow=on  InputSameDT=on  OutDataTypeStr=Inherit: Same as first input
  Real-Imag to Complex : RealImagToComplex
  Series RLC Branch : powerlib/Elements/Series RLC Branch  LConnTagsString=__new0  RConnTagsString=__new0  BranchType=R  Resistance=1e6  Inductance=1e-3  SetiL0=off  InitialCurrent=0  Capacitance=1e-6  Setx0=off  InitialVoltage=0  Measurements=None
  Series RLC Branch1 : powerlib/Elements/Series RLC Branch  LConnTagsString=__new0  RConnTagsString=__new0  BranchType=R  Resistance=1e6  Inductance=1e-3  SetiL0=off  InitialCurrent=0  Capacitance=1e-6  Setx0=off  InitialVoltage=0  Measurements=None
  Voltage Measurement1 : powerlib/Measurements/Voltage Measurement  PhasorSimulation=on  OutputType=Complex  PSBequivalent=0
  Voltage Measurement2 : powerlib/Measurements/Voltage Measurement  PhasorSimulation=on  OutputType=Complex  PSBequivalent=0
  a^2 : Gain  Gain=exp(-j*2*pi/3)  SaturateOnIntegerOverflow=on  OutDataTypeStr=Inherit: Same as input  ParamDataTypeStr=Inherit: Same as input
  "a^2 " : Gain  Gain=exp(-j*2*pi/3)  SaturateOnIntegerOverflow=on  OutDataTypeStr=Inherit: Same as input  ParamDataTypeStr=Inherit: Same as input
  a^3 : Gain  Gain=1/3  SaturateOnIntegerOverflow=on  OutDataTypeStr=Inherit: Same as input  ParamDataTypeStr=Inherit: Same as input
  a^4 : Gain  Gain=2/3  SaturateOnIntegerOverflow=on  OutDataTypeStr=Inherit: Same as input  ParamDataTypeStr=Inherit: Same as input
  A : PMIOPort  Tag=PMCPort  Port=1  Side=Right
  B : PMIOPort  Tag=PMCPort  Port=2  Side=Right
  C : PMIOPort  Tag=PMCPort  Port=3  Side=Right
  wires:
  [Ib] -> CSb/1
  Break Alg. Loop 1/1(Out) -> a^2/1, [Ia]
  a^4/1 -> Conj1/1
  "a^2 "/1 -> Add/2
  [Vbc] -> "a^2 "/1
  [Vab] -> Add/1
  Add/1 -> a^3/1
  a^3/1 -> Avoid division by zero/1(I)
  Conj1/1 -> Break Alg. Loop 1/1(In)
  Avoid division by zero/1(O) -> Product/1  "V1"
  a^2/1 -> [Ib]
  [Ia] -> Csa/1
  Product/1 -> a^4/1  "I1"
  Real-Imag to Complex/1 -> Product/2
  Voltage Measurement2/1 -> [Vbc]
  Voltage Measurement1/1 -> [Vab]
  P/1 -> Real-Imag to Complex/1
  2/1 -> Real-Imag to Complex/2
  connections:
  CSb/RConn1 -- Voltage Measurement1/LConn2 -- Voltage Measurement2/LConn1 -- Series RLC Branch/RConn1 -- B/RConn1 -- Series RLC Branch1/LConn1
  Voltage Measurement2/LConn2 -- Csa/LConn1 -- CSb/LConn1 -- C/RConn1 -- Series RLC Branch1/RConn1
  A/RConn1 -- Series RLC Branch/LConn1 -- Voltage Measurement1/LConn1 -- Csa/RConn1

== system power_V2G_GA/Power measurements/Load  Power ==
  Sum : Sum  Inputs=++++
  S : Outport
  wires:
  Sum/1 -> S/1
  [S_EV] -> Sum/2
  [S_charg] -> Sum/3
  [S_load] -> Sum/1
  [S_asm] -> Sum/4

== system power_V2G_GA/Power measurements/Load active Power1 ==
  Gain1 : Gain  Gain=-1
  Sum : Sum  Inputs=|++++
  P : Outport
  wires:
  [P_asm] -> Sum/4
  Sum/1 -> Gain1/1
  [P_charg] -> Sum/3
  [P_load] -> Sum/1
  [P_EV] -> Sum/2
  Gain1/1 -> P/1

== system power_V2G_GA/Power measurements/Load reactive Power ==
  Gain1 : Gain  Gain=-1
  Sum : Sum  Inputs=|++++
  "Q " : Outport
  wires:
  Sum/1 -> Gain1/1
  [Q_charg] -> Sum/3
  [Q_load] -> Sum/1
  [Q_EV] -> Sum/2
  Gain1/1 -> "Q "/1
  [Q_asm] -> Sum/4

== system power_V2G_GA/Scopes /ASMdata ==
  Complex to Magnitude-Angle : ComplexToMagnitudeAngle
  Complex to Magnitude-Angle1 : ComplexToMagnitudeAngle
  Demux : Demux  Outputs=1
  Demux1 : Demux  Outputs=1
  Gain : Gain  Gain=3/2
  Product : Product
  Product1 : Product
  Product2 : Product
  Scope : Scope
      settings: SaveName=ScopeData3
  Sum : Sum  Inputs=|+-
  Trigonometric Function : Trigonometry  Operator=cos
  Trigonometric Function1 : Trigonometry
  V asm : Outport
  I asm : Outport  Port=2
  S asm : Outport  Port=3
  P asm : Outport  Port=4
  Q asm : Outport  Port=5
  tag scope: P_asm=global, Q_asm=global, S_asm=global
  wires:
  Product2/1 -> Q asm/1, [Q_asm]
  Product1/1 -> P asm/1, [P_asm]
  Trigonometric Function/1 -> Product1/2
  Trigonometric Function1/1 -> Product2/2
  Sum/1 -> Trigonometric Function/1, Trigonometric Function1/1
  Complex to Magnitude-Angle/2 -> Sum/1
  [Iasm] -> Complex to Magnitude-Angle1/1
  [Vasm] -> Complex to Magnitude-Angle/1
  Complex to Magnitude-Angle1/2 -> Sum/2, Scope/1
  Product/1 -> Product1/1, Product2/1, S asm/1, [S_asm]
  Demux1/1 -> Product/2
  Gain/1 -> Product/1
  Complex to Magnitude-Angle1/1 -> Demux1/1, I asm/1
  Complex to Magnitude-Angle/1 -> Demux/1, V asm/1
  Demux/1 -> Gain/1

== system power_V2G_GA/Scopes /Charge data ==
  Complex to Magnitude-Angle : ComplexToMagnitudeAngle
  Complex to Magnitude-Angle1 : ComplexToMagnitudeAngle
  Demux : Demux  Outputs=1
  Demux1 : Demux  Outputs=1
  Gain : Gain  Gain=3/2
  Product : Product
  Product1 : Product
  Product2 : Product
  Sum : Sum  Inputs=|+-
  Trigonometric Function : Trigonometry  Operator=cos
  Trigonometric Function1 : Trigonometry
  V charg : Outport
  I charg : Outport  Port=2
  S charg : Outport  Port=3
  P charg : Outport  Port=4
  Q charg : Outport  Port=5
  tag scope: P_charg=global, Q_charg=global, S_charg=global
  wires:
  Demux/1 -> Gain/1
  Complex to Magnitude-Angle/1 -> V charg/1, Demux/1
  Complex to Magnitude-Angle1/1 -> I charg/1, Demux1/1
  Gain/1 -> Product/1
  Demux1/1 -> Product/2
  Product/1 -> [S_charg], S charg/1, Product2/1, Product1/1
  Complex to Magnitude-Angle1/2 -> Sum/2
  [V_charg] -> Complex to Magnitude-Angle/1
  [I_charg] -> Complex to Magnitude-Angle1/1
  Complex to Magnitude-Angle/2 -> Sum/1
  Sum/1 -> Trigonometric Function1/1, Trigonometric Function/1
  Trigonometric Function1/1 -> Product2/2
  Trigonometric Function/1 -> Product1/2
  Product1/1 -> [P_charg], P charg/1
  Product2/1 -> [Q_charg], Q charg/1

== system power_V2G_GA/Scopes /Load data  ==
  Complex to Magnitude-Angle : ComplexToMagnitudeAngle
  Complex to Magnitude-Angle1 : ComplexToMagnitudeAngle
  Demux : Demux  Outputs=1
  Demux1 : Demux  Outputs=1
  Gain : Gain  Gain=3/2
  Product : Product
  Product1 : Product
  Product2 : Product
  Scope : Scope  NumInputPorts=2
      settings: YMin=-3.5~0  YMax=3.5~10000  SaveName=ScopeData3
  Sum : Sum  Inputs=|+-
  Trigonometric Function : Trigonometry  Operator=cos
  Trigonometric Function1 : Trigonometry
  V load : Outport
  I load : Outport  Port=2
  S load : Outport  Port=3
  P load : Outport  Port=4
  Q load : Outport  Port=5
  tag scope: P_load=global, Q_load=global, S_load=global
  wires:
  Demux/1 -> Gain/1
  Complex to Magnitude-Angle/1 -> V load/1, Demux/1
  Complex to Magnitude-Angle1/1 -> Scope/2, I load/1, Demux1/1
  Gain/1 -> Product/1
  Demux1/1 -> Product/2
  Product/1 -> [S_load], S load/1, Product2/1, Product1/1
  Complex to Magnitude-Angle1/2 -> Scope/1, Sum/2
  [Vload] -> Complex to Magnitude-Angle/1
  [Iload] -> Complex to Magnitude-Angle1/1
  Complex to Magnitude-Angle/2 -> Sum/1
  Sum/1 -> Trigonometric Function1/1, Trigonometric Function/1
  Trigonometric Function1/1 -> Product2/2
  Trigonometric Function/1 -> Product1/2
  Product1/1 -> [P_load], P load/1
  Product2/1 -> [Q_load], Q load/1

== system power_V2G_GA/Scopes /PV farm data  ==
  Complex to Magnitude-Angle : ComplexToMagnitudeAngle
  Complex to Magnitude-Angle1 : ComplexToMagnitudeAngle
  Demux : Demux  Outputs=1
  Demux1 : Demux  Outputs=1
  Gain : Gain  Gain=3/2
  Product : Product
  Product1 : Product
  Product2 : Product
  Sum : Sum  Inputs=|+-
  Trigonometric Function : Trigonometry  Operator=cos
  Trigonometric Function1 : Trigonometry
  V PV : Outport
  I PV : Outport  Port=2
  S PV : Outport  Port=3
  P PV : Outport  Port=4
  Q PV : Outport  Port=5
  tag scope: P_PV=global, Q_PV=global, S_PV=global
  wires:
  Demux/1 -> Gain/1
  Complex to Magnitude-Angle/1 -> V PV/1, Demux/1
  Complex to Magnitude-Angle1/1 -> I PV/1, Demux1/1
  Gain/1 -> Product/1
  Demux1/1 -> Product/2
  Product/1 -> [S_PV], S PV/1, Product2/1, Product1/1
  Complex to Magnitude-Angle1/2 -> Sum/2
  [VabcPV] -> Complex to Magnitude-Angle/1
  [IabcPV] -> Complex to Magnitude-Angle1/1
  Complex to Magnitude-Angle/2 -> Sum/1
  Sum/1 -> Trigonometric Function1/1, Trigonometric Function/1
  Trigonometric Function1/1 -> Product2/2
  Trigonometric Function/1 -> Product1/2
  Product1/1 -> [P_PV], P PV/1
  Product2/1 -> [Q_PV], Q PV/1
